simulink model "test_staticCompensator"  (R2013a)
settings: Solver=ode15s  StartTime=0.0  StopTime=5  MaxStep=1e-2  RelTol=1e-5
libraries: usask_hyd_ssc_lib x5, fl_lib x5, nesl_utility x4, simulink x1
settings Model: Creator=tkw954  LastModifiedBy=tkw954
settings SolverCC: MaxConsecutiveMinStep=100
settings SimscapeCC: SimscapeLogType=all  SimscapeLogLimitData=off

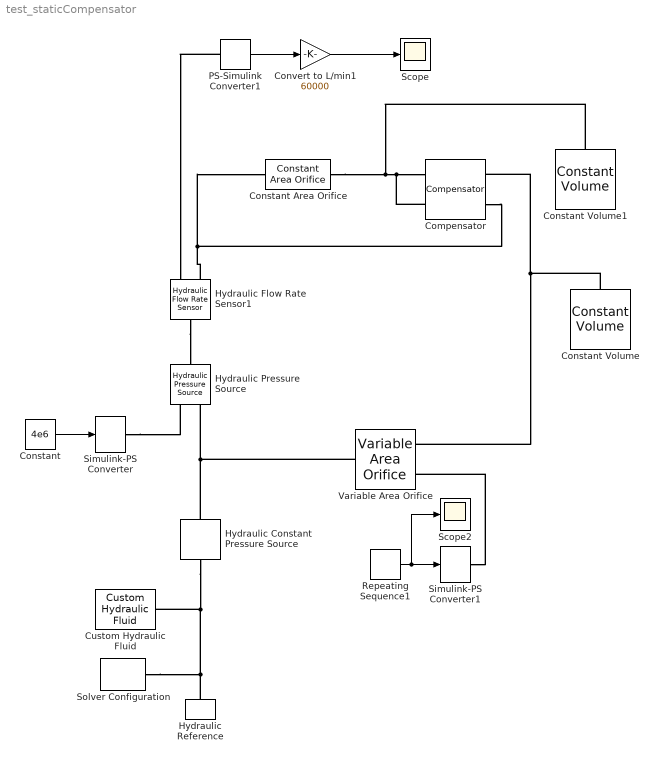
== system test_staticCompensator ==
  Compensator : usask_hyd_ssc_lib/Compensator  A1=1e-9 m^2  P1=-1.1e6 Pa  A2=25e-6 m^2  P2=-1e6 Pa  Cd=0.61  q_Log=off  dP_AB_Log=off  Pw_Log=off  Area_Log=off  LocalVarNames=|q|p|Pw  LocalVarDescs=|Volumetric flow rate|Pressure|Power Loss  LocalVarLogging=[0 0 0]
  Constant : Constant  Value=4e6
  Constant Area Orifice : usask_hyd_ssc_lib/Constant Area Orifice  A=10e-6 m^2  Cd=0.61  q_Log=off  p_Log=off  Pw_Log=off  LocalVarNames=|q|p|Pw  LocalVarDescs=|Volumetric flow rate|Pressure|Power Loss  LocalVarLogging=[0 0 0]
  Constant Volume : usask_hyd_ssc_lib/Constant Volume  V=0.1e-3 m^3  p0=0 Pa  q_Log=off  p_Log=off  LocalVarNames=|q|p  LocalVarDescs=|Flow rate into chamber|Pressure in the chamber  LocalVarLogging=[0 0]
  Constant Volume1 : usask_hyd_ssc_lib/Constant Volume  V=0.01e-3 m^3  p0=0 Pa  q_Log=off  p_Log=off  LocalVarNames=|q|p  LocalVarDescs=|Flow rate into chamber|Pressure in the chamber  LocalVarLogging=[0 0]
  Convert to L/min1 : Gain  Gain=60000
  Custom Hydraulic Fluid : fl_lib/Hydraulic/Hydraulic Utilities/Custom Hydraulic Fluid  density=850 kg/m^3  viscosity_kin=18e-6 m^2/s  bulk=0.8e9 Pa  alpha=0.005  LocalVarLogging=[]
  Hydraulic Constant Pressure Source : fl_lib/Hydraulic/Hydraulic Sources/Hydraulic Constant Pressure Source  commanded_pressure=0 Pa  pressure_Log=off  flow_rate_Log=off  power_Log=off  LocalVarNames=|pressure|flow_rate|power  LocalVarDescs=|Pressure differential|Flow rate|Power generated by the source  LocalVarLogging=[0 0 0]
  Hydraulic Flow Rate Sensor1 : fl_lib/Hydraulic/Hydraulic Sensors/Hydraulic Flow Rate Sensor  q_Log=off  p_Log=off  LocalVarNames=|q|p  LocalVarDescs=|q|p  LocalVarLogging=[0 0]
  Hydraulic Pressure Source : fl_lib/Hydraulic/Hydraulic Sources/Hydraulic Pressure Source  q_Log=off  p_Log=off  LocalVarNames=|q|p  LocalVarDescs=|q|p  LocalVarLogging=[0 0]
  Hydraulic Reference : fl_lib/Hydraulic/Hydraulic Elements/Hydraulic Reference  q_Log=off  LocalVarNames=|q  LocalVarDescs=|q  LocalVarLogging=0
  PS-Simulink Converter1 : nesl_utility/PS-Simulink Converter  PhysicalDomain=network_engine_domain  SubClassName=ps_output  LeftPortType=input  RightPortType=output  PseudoPeriodic=off  Frequencies=[]  Unit=1  AffineConversion=off
  Repeating Sequence1 : simulink/Sources/Repeating Sequence  rep_seq_t=[0 1 1.1 2 2.1 3]  rep_seq_y=10e-6+[0 0 1 1 0 0]*10e-6;
  Scope : Scope
  Scope2 : Scope
      settings: SaveName=ScopeData2
  Simulink-PS Converter : nesl_utility/Simulink-PS Converter  PhysicalDomain=network_engine_domain  SubClassName=ps_input  LeftPortType=input  RightPortType=output  PseudoPeriodic=off  Frequencies=[]  NoiseDistribution=none  NoiseParameters=[]  Unit=1  AffineConversion=off  InputFiltering=on  SimscapeFilterOrder=1  InputFilterTimeConstant=0.001  UdotUserProvided=1
  Simulink-PS Converter1 : nesl_utility/Simulink-PS Converter  PhysicalDomain=network_engine_domain  SubClassName=ps_input  LeftPortType=input  RightPortType=output  PseudoPeriodic=off  Frequencies=[]  NoiseDistribution=none  NoiseParameters=[]  Unit=1  AffineConversion=off  InputFiltering=on  SimscapeFilterOrder=1  InputFilterTimeConstant=0.001  UdotUserProvided=1
  Solver Configuration : nesl_utility/Solver Configuration  PhysicalDomain=network_engine_domain  SubClassName=solver  LeftPortType=input  RightPortType=generic  Accelerate=off  Tones=[]  Harmonics=[]  SimulateNoise=off  Profile=off  UseLocalSampling=off  EnableSwitchedLinearOptims=on  FrequencyDomain=off  UseCCode=off  UseNewInitialization=off  DoDC=off  ResidualTolerance=1e-09  UseLocalSolver=off  LocalSolverChoice=NE_BACKWARD_EULER_ADVANCER  LocalSolverSampleTime=0.001  DoFixedCost=off  MaxNonlinIter=3  MaxModeIter=2  LinearAlgebra=Sparse  DelaysMemoryBudget=1024
  Variable Area Orifice : usask_hyd_ssc_lib/Variable Area Orifice  Cd=0.61  Al=1e-9 m^2  q_Log=off  p_Log=off  Pw_Log=off  LocalVarNames=|q|p|Pw  LocalVarDescs=|Volumetric flow rate|Pressure|Power Loss  LocalVarLogging=[0 0 0]
  wires:
  PS-Simulink Converter1/1 -> Convert to L/min1/1
  Convert to L/min1/1 -> Scope/1
  Repeating Sequence1/1 -> Scope2/1, Simulink-PS Converter1/1
  Constant/1 -> Simulink-PS Converter/1
  connections:
  Hydraulic Reference/LConn1 -- Solver Configuration/RConn1 -- Hydraulic Constant Pressure Source/RConn1 -- Custom Hydraulic Fluid/RConn1
  Simulink-PS Converter/RConn1 -- Hydraulic Pressure Source/RConn1
  Hydraulic Constant Pressure Source/LConn1 -- Variable Area Orifice/RConn1 -- Hydraulic Pressure Source/RConn2
  Hydraulic Flow Rate Sensor1/LConn1 -- Hydraulic Pressure Source/LConn1
  PS-Simulink Converter1/LConn1 -- Hydraulic Flow Rate Sensor1/RConn1
  Hydraulic Flow Rate Sensor1/RConn2 -- Compensator/RConn2 -- Constant Area Orifice/LConn1
  Constant Area Orifice/RConn1 -- Constant Volume1/LConn1 -- Compensator/LConn2 -- Compensator/LConn1
  Compensator/RConn1 -- Variable Area Orifice/LConn1 -- Constant Volume/LConn1
  Simulink-PS Converter1/RConn1 -- Variable Area Orifice/LConn2
